simulink model "jointSpace_delta"  (R2018a)
settings: Solver=VariableStepAuto  StartTime=0.0  StopTime=10.0  RelTol=1e-3
values from neighbouring files (symbols this model uses):
  q0 = [0;0;0]    [HapticsSetup.m]
  qd0 = inv(deltaJacobian([q0;x0]))*xd0    [HapticsSetup.m]
  x0 = interx(p(:,1),p(:,2),p(:,3),Lb,Lb,Lb,0)    [HapticsSetup.m]
undefined symbols (not defined in the file or in its folder): Amatrix, Cmatrix, deltaJacobian, Gmatrix
settings Model: Creator=klay  LastModifiedBy=augus
settings CodeAppCC: StateflowObjectComments=on

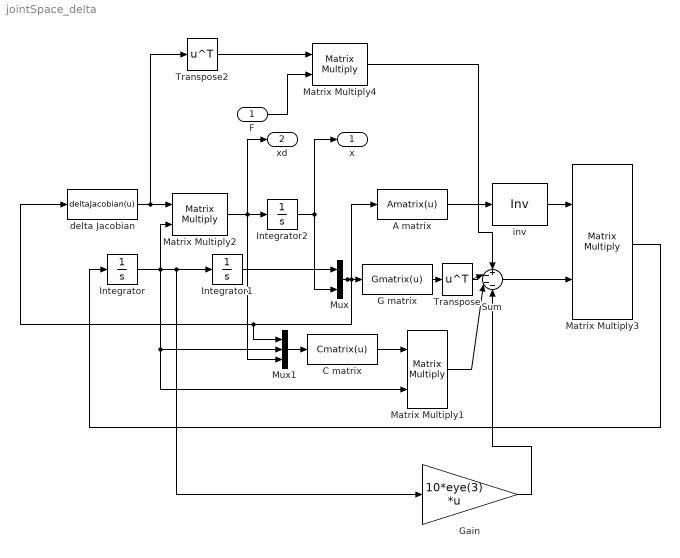
== system jointSpace_delta ==
  F : Inport  PortDimensions=3
  A matrix : MATLABFcn  MATLABFcn=Amatrix(u)  Output1D=off
  C matrix : MATLABFcn  MATLABFcn=Cmatrix(u)  Output1D=off
  G matrix : MATLABFcn  MATLABFcn=Gmatrix(u)  Output1D=off
  Gain : Gain  Gain=10*eye(3)  Multiplication=Matrix(K*u)
  Integrator : Integrator  InitialCondition=qd0
  Integrator1 : Integrator  InitialCondition=q0
  Integrator2 : Integrator  InitialCondition=x0
  Matrix Multiply{1..4} (4 alike) : Product  Multiplication=Matrix(*)
  Mux : Mux  Inputs=2
  Mux1 : Mux  Inputs=3
  Sum : Sum  Inputs=+---
  Transpose : Math  Operator=transpose  SaturateOnIntegerOverflow=on
  Transpose2 : Math  Operator=transpose  SaturateOnIntegerOverflow=on
  delta Jacobian : MATLABFcn  MATLABFcn=deltaJacobian(u)  Output1D=off
  inv : Product  Inputs=/  Multiplication=Matrix(*)
  x : Outport
  xd : Outport  Port=2
  wires:
  Integrator/1 -> Gain/1, Integrator1/1, Matrix Multiply1/2, Mux1/2, Matrix Multiply2/2
  Integrator2/1 -> x/1, Mux/2
  delta Jacobian/1 -> Transpose2/1, Matrix Multiply2/1
  Matrix Multiply2/1 -> Mux1/3, xd/1, Integrator2/1
  Mux/1 -> Mux1/1, delta Jacobian/1, A matrix/1, G matrix/1
  Integrator1/1 -> Mux/1
  Mux1/1 -> C matrix/1
  C matrix/1 -> Matrix Multiply1/1
  Matrix Multiply1/1 -> Sum/3
  Sum/1 -> Matrix Multiply3/2
  A matrix/1 -> inv/1
  inv/1 -> Matrix Multiply3/1
  Matrix Multiply3/1 -> Integrator/1
  F/1 -> Matrix Multiply4/2
  Transpose2/1 -> Matrix Multiply4/1
  Matrix Multiply4/1 -> Sum/1
  G matrix/1 -> Transpose/1
  Transpose/1 -> Sum/2
  Gain/1 -> Sum/4
